simulink model "pfb_fir_generic_async_test_sim4"  (R2012b)
settings: Solver=VariableStepDiscrete  StartTime=0.0  StopTime=10.0  RelTol=1e-3
model workspace (MAT data in the model file):
  synci = [0 1 2 3 4 5 6 7 8 9 10 11 ... (131074 elements, 65537x2)]
  din0 = [0 1 2 3 4 5 6 7 8 9 10 11 ... (16386 elements, 8193x2)]
  din1 = [0 1 2 3 4 5 6 7 8 9 10 11 ... (16386 elements, 8193x2)]
  din2 = [0 1 2 3 4 5 6 7 8 9 10 11 ... (16386 elements, 8193x2)]
  din3 = [0 1 2 3 4 5 6 7 8 9 10 11 ... (16386 elements, 8193x2)]
  din4 = [0 1 2 3 4 5 6 7 8 9 10 11 ... (16386 elements, 8193x2)]
  din5 = [0 1 2 3 4 5 6 7 8 9 10 11 ... (16386 elements, 8193x2)]
  din6 = [0 1 2 3 4 5 6 7 8 9 10 11 ... (16386 elements, 8193x2)]
  din7 = [0 1 2 3 4 5 6 7 8 9 10 11 ... (16386 elements, 8193x2)]
  dvalid = [0 1 2 3 4 5 6 7 8 9 10 11 ... (131072 elements, 65536x2)]
libraries: xbsIndex_r4 x3718, casper_library_delays x1
(part 2 of 18)

== system pfb_fir_generic_async_test_sim4/inputs ==
  din0_fw : FromWorkspace  VariableName=din0  SampleTime=1
  din0_gi : xbsIndex_r4/Gateway In  gui_display_data_type=Fixed-point  arith_type="Signed  (2's comp)"  n_bits=10  bin_pt=9  preci_type=Single  exp_width=8  frac_width=24  quantization="Round  (unbiased: +/- Inf)"  overflow=Saturate  period=1  dbl_ovrd=off  timing_constraint=None  locs_specified=off  LOCs={}  UseAsADC=off  ADCChannel='1'  inherit_from_input=off  hdl_port=on  block_type=gatewayin
  din1_fw : FromWorkspace  VariableName=din1  SampleTime=1
  din1_gi : xbsIndex_r4/Gateway In  gui_display_data_type=Fixed-point  arith_type="Signed  (2's comp)"  n_bits=10  bin_pt=9  preci_type=Single  exp_width=8  frac_width=24  quantization="Round  (unbiased: +/- Inf)"  overflow=Saturate  period=1  dbl_ovrd=off  timing_constraint=None  locs_specified=off  LOCs={}  UseAsADC=off  ADCChannel='1'  inherit_from_input=off  hdl_port=on  block_type=gatewayin
  din2_fw : FromWorkspace  VariableName=din2  SampleTime=1
  din2_gi : xbsIndex_r4/Gateway In  gui_display_data_type=Fixed-point  arith_type="Signed  (2's comp)"  n_bits=10  bin_pt=9  preci_type=Single  exp_width=8  frac_width=24  quantization="Round  (unbiased: +/- Inf)"  overflow=Saturate  period=1  dbl_ovrd=off  timing_constraint=None  locs_specified=off  LOCs={}  UseAsADC=off  ADCChannel='1'  inherit_from_input=off  hdl_port=on  block_type=gatewayin
  din3_fw : FromWorkspace  VariableName=din3  SampleTime=1
  din3_gi : xbsIndex_r4/Gateway In  gui_display_data_type=Fixed-point  arith_type="Signed  (2's comp)"  n_bits=10  bin_pt=9  preci_type=Single  exp_width=8  frac_width=24  quantization="Round  (unbiased: +/- Inf)"  overflow=Saturate  period=1  dbl_ovrd=off  timing_constraint=None  locs_specified=off  LOCs={}  UseAsADC=off  ADCChannel='1'  inherit_from_input=off  hdl_port=on  block_type=gatewayin
  din4_fw : FromWorkspace  VariableName=din4  SampleTime=1
  din4_gi : xbsIndex_r4/Gateway In  gui_display_data_type=Fixed-point  arith_type="Signed  (2's comp)"  n_bits=10  bin_pt=9  preci_type=Single  exp_width=8  frac_width=24  quantization="Round  (unbiased: +/- Inf)"  overflow=Saturate  period=1  dbl_ovrd=off  timing_constraint=None  locs_specified=off  LOCs={}  UseAsADC=off  ADCChannel='1'  inherit_from_input=off  hdl_port=on  block_type=gatewayin
  din5_fw : FromWorkspace  VariableName=din5  SampleTime=1
  din5_gi : xbsIndex_r4/Gateway In  gui_display_data_type=Fixed-point  arith_type="Signed  (2's comp)"  n_bits=10  bin_pt=9  preci_type=Single  exp_width=8  frac_width=24  quantization="Round  (unbiased: +/- Inf)"  overflow=Saturate  period=1  dbl_ovrd=off  timing_constraint=None  locs_specified=off  LOCs={}  UseAsADC=off  ADCChannel='1'  inherit_from_input=off  hdl_port=on  block_type=gatewayin
  din6_fw : FromWorkspace  VariableName=din6  SampleTime=1
  din6_gi : xbsIndex_r4/Gateway In  gui_display_data_type=Fixed-point  arith_type="Signed  (2's comp)"  n_bits=10  bin_pt=9  preci_type=Single  exp_width=8  frac_width=24  quantization="Round  (unbiased: +/- Inf)"  overflow=Saturate  period=1  dbl_ovrd=off  timing_constraint=None  locs_specified=off  LOCs={}  UseAsADC=off  ADCChannel='1'  inherit_from_input=off  hdl_port=on  block_type=gatewayin
  din7_fw : FromWorkspace  VariableName=din7  SampleTime=1
  din7_gi : xbsIndex_r4/Gateway In  gui_display_data_type=Fixed-point  arith_type="Signed  (2's comp)"  n_bits=10  bin_pt=9  preci_type=Single  exp_width=8  frac_width=24  quantization="Round  (unbiased: +/- Inf)"  overflow=Saturate  period=1  dbl_ovrd=off  timing_constraint=None  locs_specified=off  LOCs={}  UseAsADC=off  ADCChannel='1'  inherit_from_input=off  hdl_port=on  block_type=gatewayin
  dvalid_fw : FromWorkspace  VariableName=dvalid  SampleTime=1
  dvalid_gi : xbsIndex_r4/Gateway In  gui_display_data_type=Fixed-point  arith_type="Signed  (2's comp)"  n_bits=10  bin_pt=9  preci_type=Single  exp_width=8  frac_width=24  quantization="Round  (unbiased: +/- Inf)"  overflow=Saturate  period=1  dbl_ovrd=off  timing_constraint=None  locs_specified=off  LOCs={}  UseAsADC=off  ADCChannel='1'  inherit_from_input=off  hdl_port=on  block_type=gatewayin
  synci_fw : FromWorkspace  VariableName=synci  SampleTime=1
  synci_gi : xbsIndex_r4/Gateway In  gui_display_data_type=Fixed-point  arith_type=Boolean  n_bits=1  bin_pt=0  preci_type=Single  exp_width=8  frac_width=24  quantization=Truncate  overflow=Flag as error  period=1  dbl_ovrd=off  timing_constraint=None  locs_specified=off  LOCs={}  UseAsADC=off  ADCChannel='1'  inherit_from_input=off  hdl_port=on  block_type=gatewayin
  synci : Outport
  din0 : Outport  Port=2
  din1 : Outport  Port=3
  din2 : Outport  Port=4
  din3 : Outport  Port=5
  din4 : Outport  Port=6
  din5 : Outport  Port=7
  din6 : Outport  Port=8
  din7 : Outport  Port=9
  dvalid : Outport  Port=10
  wires:
  synci_fw/1 -> synci_gi/1
  synci_gi/1 -> synci/1
  din0_fw/1 -> din0_gi/1
  din1_fw/1 -> din1_gi/1
  din2_fw/1 -> din2_gi/1
  din3_fw/1 -> din3_gi/1
  din4_fw/1 -> din4_gi/1
  din5_fw/1 -> din5_gi/1
  din6_fw/1 -> din6_gi/1
  din7_fw/1 -> din7_gi/1
  din0_gi/1 -> din0/1
  din1_gi/1 -> din1/1
  din2_gi/1 -> din2/1
  din3_gi/1 -> din3/1
  din4_gi/1 -> din4/1
  din5_gi/1 -> din5/1
  din6_gi/1 -> din6/1
  din7_gi/1 -> din7/1
  dvalid_fw/1 -> dvalid_gi/1
  dvalid_gi/1 -> dvalid/1

== system pfb_fir_generic_async_test_sim4/outputs ==
  synco : Inport
  dout0 : Inport  Port=2
  dout1 : Inport  Port=3
  dout2 : Inport  Port=4
  dout3 : Inport  Port=5
  dout4 : Inport  Port=6
  dout5 : Inport  Port=7
  dout6 : Inport  Port=8
  dout7 : Inport  Port=9
  dout8 : Inport  Port=10
  dout0_go : xbsIndex_r4/Gateway Out  inherit_from_input=off  hdl_port=on  timing_constraint=None  locs_specified=off  LOCs={}  UseAsDAC=off  DACChannel='1'  block_type=gatewayout
  dout0_ri : xbsIndex_r4/Reinterpret  force_arith_type=on  arith_type="Signed  (2's comp)"  force_bin_pt=on  bin_pt=17  block_type=reinterpret
  dout0_tw : ToWorkspace  VariableName=dout0
  dout1_go : xbsIndex_r4/Gateway Out  inherit_from_input=off  hdl_port=on  timing_constraint=None  locs_specified=off  LOCs={}  UseAsDAC=off  DACChannel='1'  block_type=gatewayout
  dout1_ri : xbsIndex_r4/Reinterpret  force_arith_type=on  arith_type="Signed  (2's comp)"  force_bin_pt=on  bin_pt=17  block_type=reinterpret
  dout1_tw : ToWorkspace  VariableName=dout1
  dout2_go : xbsIndex_r4/Gateway Out  inherit_from_input=off  hdl_port=on  timing_constraint=None  locs_specified=off  LOCs={}  UseAsDAC=off  DACChannel='1'  block_type=gatewayout
  dout2_ri : xbsIndex_r4/Reinterpret  force_arith_type=on  arith_type="Signed  (2's comp)"  force_bin_pt=on  bin_pt=17  block_type=reinterpret
  dout2_tw : ToWorkspace  VariableName=dout2
  dout3_go : xbsIndex_r4/Gateway Out  inherit_from_input=off  hdl_port=on  timing_constraint=None  locs_specified=off  LOCs={}  UseAsDAC=off  DACChannel='1'  block_type=gatewayout
  dout3_ri : xbsIndex_r4/Reinterpret  force_arith_type=on  arith_type="Signed  (2's comp)"  force_bin_pt=on  bin_pt=17  block_type=reinterpret
  dout3_tw : ToWorkspace  VariableName=dout3
  dout4_go : xbsIndex_r4/Gateway Out  inherit_from_input=off  hdl_port=on  timing_constraint=None  locs_specified=off  LOCs={}  UseAsDAC=off  DACChannel='1'  block_type=gatewayout
  dout4_ri : xbsIndex_r4/Reinterpret  force_arith_type=on  arith_type="Signed  (2's comp)"  force_bin_pt=on  bin_pt=17  block_type=reinterpret
  dout4_tw : ToWorkspace  VariableName=dout4
  dout5_go : xbsIndex_r4/Gateway Out  inherit_from_input=off  hdl_port=on  timing_constraint=None  locs_specified=off  LOCs={}  UseAsDAC=off  DACChannel='1'  block_type=gatewayout
  dout5_ri : xbsIndex_r4/Reinterpret  force_arith_type=on  arith_type="Signed  (2's comp)"  force_bin_pt=on  bin_pt=17  block_type=reinterpret
  dout5_tw : ToWorkspace  VariableName=dout5
  dout6_go : xbsIndex_r4/Gateway Out  inherit_from_input=off  hdl_port=on  timing_constraint=None  locs_specified=off  LOCs={}  UseAsDAC=off  DACChannel='1'  block_type=gatewayout
  dout6_ri : xbsIndex_r4/Reinterpret  force_arith_type=on  arith_type="Signed  (2's comp)"  force_bin_pt=on  bin_pt=17  block_type=reinterpret
  dout6_tw : ToWorkspace  VariableName=dout6
  dout7_go : xbsIndex_r4/Gateway Out  inherit_from_input=off  hdl_port=on  timing_constraint=None  locs_specified=off  LOCs={}  UseAsDAC=off  DACChannel='1'  block_type=gatewayout
  dout7_ri : xbsIndex_r4/Reinterpret  force_arith_type=on  arith_type="Signed  (2's comp)"  force_bin_pt=on  bin_pt=17  block_type=reinterpret
  dout7_tw : ToWorkspace  VariableName=dout7
  dvalid_go : xbsIndex_r4/Gateway Out  inherit_from_input=off  hdl_port=on  timing_constraint=None  locs_specified=off  LOCs={}  UseAsDAC=off  DACChannel='1'  block_type=gatewayout
  dvalid_ri : xbsIndex_r4/Reinterpret  force_arith_type=on  arith_type=Unsigned  force_bin_pt=on  bin_pt=0  block_type=reinterpret
  dvalid_tw : ToWorkspace  VariableName=dvalid
  synco_go : xbsIndex_r4/Gateway Out  inherit_from_input=off  hdl_port=on  timing_constraint=None  locs_specified=off  LOCs={}  UseAsDAC=off  DACChannel='1'  block_type=gatewayout
  synco_slice : xbsIndex_r4/Slice  nbits=1  boolean_output=on  mode=Upper Bit Location + Width  bit1=0  base1=MSB of Input  bit0=0  base0=LSB of Input  dbl_ovrd=off  block_type=slice
  synco_tw : ToWorkspace  VariableName=synco
  wires:
  synco_slice/1 -> synco_go/1
  synco_go/1 -> synco_tw/1
  synco/1 -> synco_slice/1
  dout0_ri/1 -> dout0_go/1
  dout0_go/1 -> dout0_tw/1
  dout1_ri/1 -> dout1_go/1
  dout1_go/1 -> dout1_tw/1
  dout2_ri/1 -> dout2_go/1
  dout2_go/1 -> dout2_tw/1
  dout3_ri/1 -> dout3_go/1
  dout3_go/1 -> dout3_tw/1
  dout4_ri/1 -> dout4_go/1
  dout4_go/1 -> dout4_tw/1
  dout5_ri/1 -> dout5_go/1
  dout5_go/1 -> dout5_tw/1
  dout6_ri/1 -> dout6_go/1
  dout6_go/1 -> dout6_tw/1
  dout7_ri/1 -> dout7_go/1
  dout7_go/1 -> dout7_tw/1
  dout0/1 -> dout0_ri/1
  dout1/1 -> dout1_ri/1
  dout2/1 -> dout2_ri/1
  dout3/1 -> dout3_ri/1
  dout4/1 -> dout4_ri/1
  dout5/1 -> dout5_ri/1
  dout6/1 -> dout6_ri/1
  dout7/1 -> dout7_ri/1
  dvalid_ri/1 -> dvalid_go/1
  dvalid_go/1 -> dvalid_tw/1
  dout8/1 -> dvalid_ri/1

== system pfb_fir_generic_async_test_sim4/pfb_fir_generic ==
  note: sync_tp1 and dval_tp1 inline
  note: 2nd mod: conv_latency -1
  note: 1st mod: conv_latency -2
  note: Modified
      | Orig: conv_latency
  note: Modified
      | Orig: conv_latency
  note: 2nd mod: conv_latency -1
  note: 1st mod: conv_latency -2
  note: sync_tp2 trails dval_tp2 by 1
  sync : Inport
  pol0_in0 : Inport  Port=2
  pol0_in1 : Inport  Port=3
  pol0_in2 : Inport  Port=4
  pol0_in3 : Inport  Port=5
  pol0_in4 : Inport  Port=6
  pol0_in5 : Inport  Port=7
  pol0_in6 : Inport  Port=8
  pol0_in7 : Inport  Port=9
  pol1_in0 : Inport  Port=10
  pol1_in1 : Inport  Port=11
  pol1_in2 : Inport  Port=12
  pol1_in3 : Inport  Port=13
  pol1_in4 : Inport  Port=14
  pol1_in5 : Inport  Port=15
  pol1_in6 : Inport  Port=16
  pol1_in7 : Inport  Port=17
  en : Inport  Port=18
  bus_convert : Subsystem  AncestorBlock=casper_library_bus/bus_convert  mask(bus_convert){n_bits_in=[31 31 31 31 31 31 31 31 31 31 31 31 31 31 31 31], bin_pt_in=27, cmplx=off, n_bits_out=18, bin_pt_out=17, quantization=1, overflow=0, latency=6, of=off, misc=off}
      mask prompts: n_bits_in "input bit widths"; bin_pt_in "input binary points"; cmplx "input complex"; n_bits_out "output bit widths"; bin_pt_out "output binary points"; quantization "quantization strategy (Truncate=0, Round  (unbiased: +/- Inf)=1, Round (unbiased: Even Values)=2)"; overflow "overflow strategy (Wrap=0, Saturate=1, Flag as error=2)"; of "overflow indication"; misc "misc support"
      mask help: Convert components of busses
      mask init:
      | bus_convert_init(gcb, ...
      |     'n_bits_in', n_bits_in, ...
      |     'bin_pt_in', bin_pt_in, ...
      |     'cmplx', cmplx, ...
      |     'n_bits_out', n_bits_out, ...
      |     'bin_pt_out', bin_pt_out, ...
      |     'quantization', quantization, ...
      |     'overflow', overflow, ...
      |     'latency', latency, ...
      |     'misc', misc, ...
      |     'of', of);
  bus_create : Subsystem  AncestorBlock=casper_library_flow_control/bus_create  mask(bus_create){inputNum=16}
      mask prompts: inputNum "Number of inputs:"
      mask init:
      | bus_create_init(gcb,...
      |     'inputNum', inputNum);
  bus_expand : Subsystem  AncestorBlock=casper_library_flow_control/bus_expand  mask(bus_expand){mode=divisions of equal size, outputNum=16, outputWidth=18, outputBinaryPt=17, outputArithmeticType=1, show_format=off, outputToWorkspace=on, variablePrefix=pfb_fir_taps_dout, outputToModelAsWell=on}
      mask prompts: outputNum "Number of outputs:"; outputWidth "Output width:"; outputBinaryPt "Output binary point position:"; outputArithmeticType "Output arithmetic type (ufix=0, fix=1, bool=2):"; show_format "Print format string?"; outputToWorkspace "Output to workspace?"; variablePrefix "Variable name prefix:"; outputToModelAsWell "Output to model as well?"
      mask help:
      | Expands a 'bus' made using a bus_create or Xilinx
      | concat block.
      | The input will be divided into the specified number
      | of outputs with the specified arithmetic types.
      | Divisions are made from most significant bit.
      mask init:
      | bus_expand_init(gcb,...
      |     'mode', mode, ...
      |     'outputNum', outputNum, ...
      |     'outputWidth', outputWidth, ...
      |     'outputBinaryPt', outputBinaryPt, ...
      |     'outputArithmeticType', outputArithmeticType, ...
      |     'show_format', show_format, ...
      |     'outputToWorkspace', outputToWorkspace, ...
      |     'variablePrefix', variablePrefix, ...
      |     'outputToModelAsWell', outputToModelAsWell);
      settings: AttributesFormatString=16 outputs, pfb_fir_taps_dout_?
      mask TypeOptions mode: divisions of equal size | divisions of arbitrary size
      mask Callback mode: bus_expand_callback();
      mask Callback outputWidth: bus_expand_callback();
      mask Callback outputToWorkspace: bus_expand_callback();
  bus_scale : Subsystem  AncestorBlock=casper_library_bus/bus_scale  mask(bus_scale){n_bits_in=[31 31 31 31 31 31 31 31 31 31 31 31 31 31 31 31], bin_pt_in=26, type_in=1, cmplx=off, scale_factor=-1, misc=off}
      mask prompts: n_bits_in "input bit widths"; bin_pt_in "input binary points"; type_in "input types"; cmplx "input complex"; scale_factor "scale factor (2^?)"; misc "misc support"
      mask help: Convert components of busses
      mask init:
      | bus_scale_init(gcb, ...
      |     'n_bits_in', n_bits_in, ...
      |     'bin_pt_in', bin_pt_in, ...
      |     'type_in', type_in, ...
      |     'cmplx', cmplx, ...
      |     'scale_factor', scale_factor, ...
      |     'misc', misc);
  coeff_munge : Subsystem  AncestorBlock=casper_library_flow_control/munge  mask(munge){divisions=64, div_size=[18 18 18 18 18 18 18 18 18 18 18 18 18 18 18 18 18 18 18 18 18 18 18 18 18 18 18 18 18 18 18 18 18 18 18 18 18 18 18 18 18 18 18 18 18 18 18 18 18 18 18 18 18 18 18 18 18 18 18 18 18 18 18 18], order=[56 56 57 57 58 58 59 59 60 60 61 61 62 62 63 63 48 48 49 49 50 50 51 51 52 52 53 53 54 54 55 55 40 40 41 41 42 42 43 43 44 44 45 45 46 46 47 47 32 32 33 33 34 34 35 35 36 36 37 37 38 38 39 39 24 24 25 25 26 26 27 27 28 28 29 29 30 30 31 31 16 16 17 17 18 18 19 19 20 20 21 21 22 22 23 23 8 8 9 9 10 10 11 11 12 12 13 13 14 14 15 15 0 0 1 1 2 2 3 3 4 4 5 5 6 6 7 7], arith_type_out=Unsigned, bin_pt_out=0}
      mask prompts: divisions "Number of divisions"; div_size "Division size (bits)"; order "Division packing order"; arith_type_out "Output arithmetic type"; bin_pt_out "Output binary point"
      mask help: Splits an input bus into the specified number of divisions and then recombines them in the order specified (most significant division = 0,least = number divisions-1)
      mask init:
      | munge_init(gcb, ...
      |     'divisions', divisions, ...
      |     'div_size', div_size, ...
      |     'order', order, ...
      |     'arith_type_out', arith_type_out, ...
      |     'bin_pt_out', bin_pt_out);
      settings: AttributesFormatString=|
      | split:[18 18 18 18 18 18 18 18 18 18 18 18 18 18 18 18 18 18 18 18 18 18 18 18 18 18 18 18 18 18 18 18 18 18 18 18 18 18 18 18 18 18 18 18 18 18 18 18 18 18 18 18 18 18 18 18 18 18 18 18 18 18 18 18]
      | join:[56 56 57 57 58 58 59 59 60 60 61 61 62 62 63 63 48 48 49 49 50 50 51 51 52 52 53 53 54 54 55 55 40 40 41 41 42 42 43 43 44 44 45 45 46 46 47 47 32 32 33 33 34 34 35 35 36 36 37 37 38 38 39 39 24 24 25 25 26 26 27 27 28 28 29 29 30 30 31 31 16 16 17 17 18 18 19 19 20 20 21 21 22 22 23 23 8 8 9 9 10 10 11 11 12 12 13 13 14 14 15 15 0 0 1 1 2 2 3 3 4 4 5 5 6 6 7 7]
      | Unsigned [2304,0]
      mask TypeOptions arith_type_out: Unsigned | Signed  (2's comp) | Floating-point
  den : xbsIndex_r4/Delay  rst=off  infoeditControl=Selection of Reset will increase slice count due to use of real FFs and instead of SRLs  en=off  latency=conv_latency  dbl_ovrd=off  reg_retiming=on  block_type=delay
  pfb_fir_coeff_gen : Subsystem  AncestorBlock=casper_library_pfbs/pfb_fir_coeff_gen  mask(pfb_fir_coeff_gen){pfb_size=13, n_taps=8, n_bits_coeff=18, WindowType=hamming, n_inputs=3, fwidth=1, async=on, bram_latency=8, fan_latency=9, add_latency=6, bram_optimization=Speed}
      mask prompts: pfb_size "Size of PFB: (2^? pnts)"; n_taps "Total Number of Taps:"; n_bits_coeff "Bitwidth of Coefficients:"; WindowType "Windowing Function:"; n_inputs "Number of Simultaneous Inputs: (2^?)"; fwidth "Bin Width (normal=1)"; async "Asynchronous operation"; bram_latency "BRAM Latency"; fan_latency "Fanout latency"; add_latency "Add latency"; bram_optimization "BRAM optimization"
      mask init:
      | pfb_fir_coeff_gen_init(gcb, ...
      |     'n_inputs', n_inputs, ...
      |     'pfb_size', pfb_size, ...
      |     'n_taps', n_taps, ...
      |     'n_bits_coeff', n_bits_coeff, ...
      |     'WindowType', WindowType, ...
      |     'fwidth', fwidth, ...
      |     'async', async, ...
      |     'bram_latency', bram_latency, ...
      |     'fan_latency', fan_latency, ...
      |     'add_latency', add_latency, ...
      |     'bram_optimization', bram_optimization);
      mask TypeOptions WindowType: bartlett | barthannwin | blackman | blackmanharris | bohamwin | chebwin | flattopwin | gausswin | hamming | hann | kaiser | nuttallwin | parzenwin | rectwin | tukeywin | triang | userwindow
      mask TypeOptions bram_optimization: Area | Speed
  pfb_fir_taps : Subsystem  AncestorBlock=casper_library_pfbs/pfb_fir_taps  mask(pfb_fir_taps){n_streams=2, n_inputs=3, pfb_size=13, n_taps=8, n_bits_data=10, n_bits_coeff=18, bin_pt_coeff=17, complex=off, async=on, mult_latency=8, add_latency=6, bram_latency=8, fan_latency=9, multiplier_implementation=behavioral HDL, bram_optimization=Speed}
      mask prompts: n_streams "Number simultaneous streams"; n_inputs "Number simultaneous inputs per stream (2^?)"; pfb_size "PFB size (2^? pnts)"; n_taps "Number of taps"; n_bits_data "Data bit width in"; n_bits_coeff "Coefficient bit width"; bin_pt_coeff "Coefficient binary point"; complex "Complex input data"; async "Asynchronous operation"; mult_latency "Multiplier latency"; add_latency "Adder latency"; bram_latency "BRAM latency"; fan_latency "Fanout latency"; multiplier_implementation "Multiplier implementation"; bram_optimization "BRAM optimization"
      mask init:
      | pfb_fir_taps_init(gcb, ...
      |     'n_streams', n_streams, ...
      |     'n_inputs', n_inputs, ...
      |     'pfb_size', pfb_size, ...
      |     'n_taps', n_taps, ...
      |     'n_bits_data', n_bits_data, ...
      |     'n_bits_coeff', n_bits_coeff, ...
      |     'bin_pt_coeff', bin_pt_coeff, ...
      |     'complex', complex, ...
      |     'async', async, ...
      |     'mult_latency', mult_latency, ...
      |     'add_latency', add_latency, ...
      |     'bram_latency', bram_latency, ...
      |     'fan_latency', fan_latency, ...
      |     'multiplier_implementation', multiplier_implementation, ...
      |     'bram_optimization', bram_optimization);
      mask TypeOptions multiplier_implementation: behavioral HDL | standard core | embedded multiplier core
      mask TypeOptions bram_optimization: Area | Speed
  sync_delay : xbsIndex_r4/Delay  rst=off  infoeditControl=Selection of Reset will increase slice count due to use of real FFs and instead of SRLs  en=off  latency=conv_latency  dbl_ovrd=off  reg_retiming=on  block_type=delay
  sync_out : Outport
  pol0_out0 : Outport  Port=2
  pol0_out1 : Outport  Port=3
  pol0_out2 : Outport  Port=4
  pol0_out3 : Outport  Port=5
  pol0_out4 : Outport  Port=6
  pol0_out5 : Outport  Port=7
  pol0_out6 : Outport  Port=8
  pol0_out7 : Outport  Port=9
  pol1_out0 : Outport  Port=10
  pol1_out1 : Outport  Port=11
  pol1_out2 : Outport  Port=12
  pol1_out3 : Outport  Port=13
  pol1_out4 : Outport  Port=14
  pol1_out5 : Outport  Port=15
  pol1_out6 : Outport  Port=16
  pol1_out7 : Outport  Port=17
  dvalid : Outport  Port=18
  wires:
  pol0_in0/1 -> bus_create/1(in1)
  bus_expand/1(msb_out16) -> pol0_out0/1
  pol0_in1/1 -> bus_create/3(in3)
  bus_expand/3(out14) -> pol0_out1/1
  pol0_in2/1 -> bus_create/5(in5)
  bus_expand/5(out12) -> pol0_out2/1
  pol0_in3/1 -> bus_create/7(in7)
  bus_expand/7(out10) -> pol0_out3/1
  pol0_in4/1 -> bus_create/9(in9)
  bus_expand/9(out8) -> pol0_out4/1
  pol0_in5/1 -> bus_create/11(in11)
  bus_expand/11(out6) -> pol0_out5/1
  pol0_in6/1 -> bus_create/13(in13)
  bus_expand/13(out4) -> pol0_out6/1
  pol0_in7/1 -> bus_create/15(in15)
  bus_expand/15(out2) -> pol0_out7/1
  pol1_in0/1 -> bus_create/2(in2)
  bus_expand/2(out15) -> pol1_out0/1
  pol1_in1/1 -> bus_create/4(in4)
  bus_expand/4(out13) -> pol1_out1/1
  pol1_in2/1 -> bus_create/6(in6)
  bus_expand/6(out11) -> pol1_out2/1
  pol1_in3/1 -> bus_create/8(in8)
  bus_expand/8(out9) -> pol1_out3/1
  pol1_in4/1 -> bus_create/10(in10)
  bus_expand/10(out7) -> pol1_out4/1
  pol1_in5/1 -> bus_create/12(in12)
  bus_expand/12(out5) -> pol1_out5/1
  pol1_in6/1 -> bus_create/14(in14)
  bus_expand/14(out3) -> pol1_out6/1
  pol1_in7/1 -> bus_create/16(in16)
  bus_expand/16(lsb_out1) -> pol1_out7/1
  bus_create/1(bus_out) -> pfb_fir_coeff_gen/2(din)
  pfb_fir_coeff_gen/3(coeffs) -> coeff_munge/1(din)
  pfb_fir_coeff_gen/2(dout) -> pfb_fir_taps/2(din)
  coeff_munge/1(dout) -> pfb_fir_taps/3(coeffs)
  pfb_fir_taps/2(dout) -> bus_scale/1(din)
  bus_scale/1(dout) -> bus_convert/1(din)
  bus_convert/1(dout) -> bus_expand/1(bus_in)
  sync/1 -> pfb_fir_coeff_gen/1(sync)
  pfb_fir_coeff_gen/1(sync_out) -> pfb_fir_taps/1(sync)
  pfb_fir_taps/1(sync_out) -> sync_delay/1
  sync_delay/1 -> sync_out/1
  en/1 -> pfb_fir_coeff_gen/3(en)
  pfb_fir_coeff_gen/4(dvalid) -> pfb_fir_taps/4(en)
  pfb_fir_taps/3(dvalid) -> den/1
  den/1 -> dvalid/1
